simulink model "openloop2wp"  (R2017b)
settings: Solver=VariableStepAuto  StartTime=0.0  StopTime=0.3  RelTol=1e-3
libraries: simulink_extras x4
settings Model: Creator=Iman  LastModifiedBy=Iman

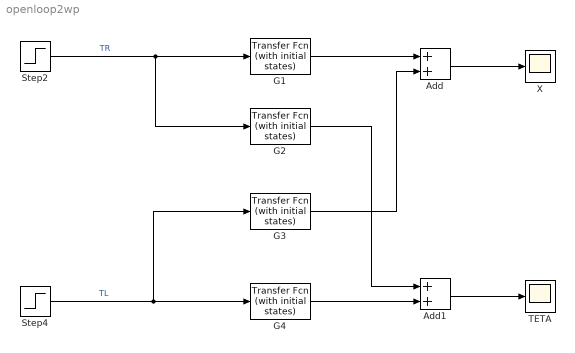
== system openloop2wp ==
  Add : Sum
  Add1 : Sum
  G1 : simulink_extras/Additional Linear/Transfer Fcn (with initial states)  N=[104.5 -3064 -6898]  D=[1 2549 -370.1 -1.285e05 0]  X0=0
  G2 : simulink_extras/Additional Linear/Transfer Fcn (with initial states)  N=[-1374 -7.66e04]  D=[1 2549 -370.1 -1.285e05]  X0=0
  G3 : simulink_extras/Additional Linear/Transfer Fcn (with initial states)  N=[104.5 -3064 -6898]  D=[1 2549 -370.1 -1.285e05 0]  X0=0
  G4 : simulink_extras/Additional Linear/Transfer Fcn (with initial states)  N=[-1374 -7.66e04]  D=[1 2549 -370.1 -1.285e05]  X0=0
  Step2 : Step  Time=0  SampleTime=0.1
  Step4 : Step  Time=0  SampleTime=0.1
  TETA : Scope
  X : Scope
  wires:
  Add/1 -> X/1
  G4/1 -> Add1/2
  Add1/1 -> TETA/1
  Step2/1 -> G2/1, G1/1  "TR"
  G2/1 -> Add1/1
  G3/1 -> Add/2
  G1/1 -> Add/1
  Step4/1 -> G3/1, G4/1  "TL"
